simulink model "irp_2018b"  (R2018b)
settings: Solver=VariableStepAuto  StartTime=0.0  StopTime=inf  RelTol=1e-3
libraries: simulink x10, simulink_extras x8
settings Model: Creator=Bartlomiej Mroz  LastModifiedBy=Bartlomiej Mroz

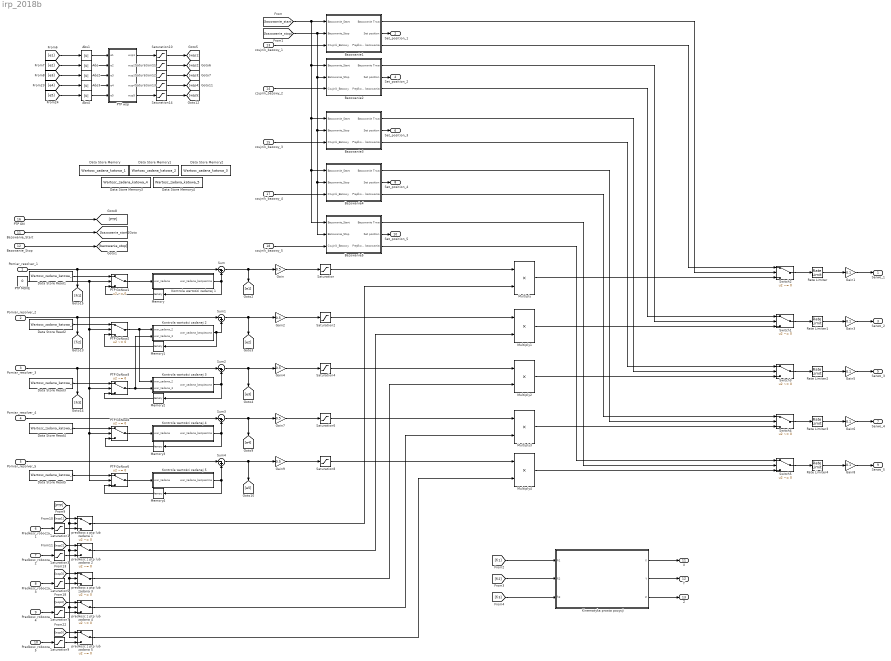
== system irp_2018b ==
  Pomiar_resolver_1 : Inport
  Pomiar_resolver_2 : Inport  Port=2
  Pomiar_resolver_3 : Inport  Port=3
  Pomiar_resolver_4 : Inport  Port=4
  Pomiar_resolver_5 : Inport  Port=5
  Predkosc_robocza_1 : Inport  Port=6
  Predkosc_robocza_2 : Inport  Port=7
  Predkosc_robocza_3 : Inport  Port=8
  Predkosc_robocza_4 : Inport  Port=9
  Predkosc_robocza_5 : Inport  Port=10
  Bazowanie_Start : Inport  Port=11
  Bazowanie_Stop : Inport  Port=12
  czujnik_bazowy_1 : Inport  Port=13
  czujnik_bazowy_2 : Inport  Port=14
  czujnik_bazowy_3 : Inport  Port=15
  PTP ON : Inport  Port=16
  czujnik_bazowy_4 : Inport  Port=17
  czujnik_bazowy_5 : Inport  Port=18
  Abs{,1..4} (5 alike) : Abs
  Bazowanie1 : Subsystem
  Bazowanie2 : Subsystem
  Bazowanie3 : Subsystem
  Bazowanie4 : Subsystem
  Bazowanie5 : Subsystem
  Data Store Memory : DataStoreMemory  DataStoreName=Wartosc_zadana_katowa_1  ReadBeforeWriteMsg=warning  WriteAfterWriteMsg=warning  WriteAfterReadMsg=warning  ShowAdditionalParam=off
  Data Store Memory1 : DataStoreMemory  DataStoreName=Wartosc_zadana_katowa_2  ReadBeforeWriteMsg=warning  WriteAfterWriteMsg=warning  WriteAfterReadMsg=warning  ShowAdditionalParam=off
  Data Store Memory2 : DataStoreMemory  DataStoreName=Wartosc_zadana_katowa_3  ReadBeforeWriteMsg=warning  WriteAfterWriteMsg=warning  WriteAfterReadMsg=warning  ShowAdditionalParam=off
  Data Store Memory3 : DataStoreMemory  DataStoreName=Wartosc_zadana_katowa_4  ReadBeforeWriteMsg=warning  WriteAfterWriteMsg=warning  WriteAfterReadMsg=warning  ShowAdditionalParam=off
  Data Store Memory4 : DataStoreMemory  DataStoreName=Wartosc_zadana_katowa_5  ReadBeforeWriteMsg=warning  WriteAfterWriteMsg=warning  WriteAfterReadMsg=warning  ShowAdditionalParam=off
  Data Store Read1 : DataStoreRead  DataStoreName=Wartosc_zadana_katowa_1
  Data Store Read2 : DataStoreRead  DataStoreName=Wartosc_zadana_katowa_2
  Data Store Read3 : DataStoreRead  DataStoreName=Wartosc_zadana_katowa_3
  Data Store Read4 : DataStoreRead  DataStoreName=Wartosc_zadana_katowa_4
  Data Store Read5 : DataStoreRead  DataStoreName=Wartosc_zadana_katowa_5
  Gain{,2,4,7,9} (5 alike) : Gain  Gain=0.5
  Gain{1,3,5..6,8} (5 alike) : Gain  Gain=0.1
  Kinematyka prosta pozycji : Subsystem
  "Kontrola wartości zadanej 1 " : Subsystem
  Kontrola wartości zadanej 2 : Subsystem
  Kontrola wartości zadanej 3 : Subsystem
  Kontrola wartości zadanej 4 : Subsystem
  Kontrola wartości zadanej 5 : Subsystem
  Memory{,1..4} (5 alike) : Memory
  Multiply{,1..4} (5 alike) : Product
  PTP GoNow{1..5} (5 alike) : Switch  Criteria=u2 ~= 0
  PTP MOVE : Constant  Value=0
  "PTP wsp " : MATLAB Function  TreatAsAtomicUnit=on
  Rate Limiter{,1..4} (5 alike) : RateLimiter  RisingSlewLimit=50  FallingSlewLimit=-50  SampleTimeMode=inherited
  Saturation{,2,4,6,8} (5 alike) : Saturate  UpperLimit=3  LowerLimit=-3
  Saturation{1,3,5,7,9} (5 alike) : Saturate  UpperLimit=1  LowerLimit=0.05
  Saturation{10..14} (5 alike) : Saturate  UpperLimit=1  LowerLimit=0
  Sum{,1..4} (5 alike) : Sum  Inputs=|-+
  Switch{1..5} (5 alike) : Switch  Criteria=u2 ~= 0
  predkosc z ptp lub zadana {1..5} (5 alike) : Switch  Criteria=u2 ~= 0
  Serwo_1 : Outport
  Set_position_1 : Outport  Port=2  VectorParamsAs1DForOutWhenUnconnected=on
  Serwo_2 : Outport  Port=3
  Set_position_2 : Outport  Port=4  VectorParamsAs1DForOutWhenUnconnected=on
  Serwo_3 : Outport  Port=5
  Set_position_3 : Outport  Port=6  VectorParamsAs1DForOutWhenUnconnected=on
  Serwo_4 : Outport  Port=7
  Set_position_4 : Outport  Port=8  VectorParamsAs1DForOutWhenUnconnected=on
  Serwo_5 : Outport  Port=9
  Set_position_5 : Outport  Port=10  VectorParamsAs1DForOutWhenUnconnected=on
  X : Outport  Port=11
  Y : Outport  Port=12
  Z : Outport  Port=13
  wires:
  Pomiar_resolver_1/1 -> Sum/1, [fi1]
  PTP GoNow1/1 -> "Kontrola wartości zadanej 1 "/1(war_zadana)
  "Kontrola wartości zadanej 1 "/1(war_zadana_bezpieczna) -> Sum/2, Memory/1
  Memory/1 -> PTP GoNow1/3
  Data Store Read1/1 -> PTP GoNow1/1
  Sum/1 -> Gain/1, [e1]
  Gain/1 -> Saturation/1
  Rate Limiter/1 -> Gain1/1
  Gain1/1 -> Serwo_1/1
  Saturation/1 -> Multiply/1
  Predkosc_robocza_1/1 -> Saturation1/1
  Bazowanie1/2("Set position ") -> Set_position_1/1
  Multiply/1 -> Switch2/3
  Bazowanie1/1("Bazowanie Trwa ") -> Switch2/2
  Bazowanie1/3(Prędkość bazowania) -> Switch2/1
  Switch2/1 -> Rate Limiter/1
  Bazowanie_Start/1 -> [bazowanie_start]
  Bazowanie_Stop/1 -> [bazowanie_stop]
  [bazowanie_start] -> Bazowanie5/1(Bazowanie_Start), Bazowanie4/1(Bazowanie_Start), Bazowanie3/1(Bazowanie_Start), Bazowanie2/1(Bazowanie_Start), Bazowanie1/1(Bazowanie_Start)
  [bazowanie_stop] -> Bazowanie5/2("Bazowanie_Stop "), Bazowanie4/2("Bazowanie_Stop "), Bazowanie3/2("Bazowanie_Stop "), Bazowanie2/2("Bazowanie_Stop "), Bazowanie1/2("Bazowanie_Stop ")
  czujnik_bazowy_1/1 -> Bazowanie1/3(Czujnik_Bazowy)
  Pomiar_resolver_2/1 -> [fi2], Sum1/1
  czujnik_bazowy_2/1 -> Bazowanie2/3(Czujnik_Bazowy)
  Saturation3/1 -> predkosc z ptp lub zadana 2/3
  Bazowanie2/3(Prędkość bazowania) -> Switch1/1
  Bazowanie2/1("Bazowanie Trwa ") -> Switch1/2
  Predkosc_robocza_2/1 -> Saturation3/1
  Saturation2/1 -> Multiply1/1
  Multiply1/1 -> Switch1/3
  Switch1/1 -> Rate Limiter1/1
  Sum1/1 -> [e2], Gain2/1
  Gain3/1 -> Serwo_2/1
  Kontrola wartości zadanej 2/1(war_zadana_bezpieczna) -> Sum1/2, Memory1/1
  Memory1/1 -> PTP GoNow2/3
  Gain2/1 -> Saturation2/1
  Data Store Read2/1 -> PTP GoNow2/1
  PTP GoNow2/1 -> Kontrola wartości zadanej 3/1(war_zadana_2), Kontrola wartości zadanej 2/1(war_zadana_2)
  Rate Limiter1/1 -> Gain3/1
  Bazowanie2/2("Set position ") -> Set_position_2/1
  Bazowanie3/3(Prędkość bazowania) -> Switch3/1
  Bazowanie3/1("Bazowanie Trwa ") -> Switch3/2
  Saturation4/1 -> Multiply2/1
  Rate Limiter2/1 -> Gain5/1
  PTP GoNow3/1 -> Kontrola wartości zadanej 3/2(war_zadana_3), Kontrola wartości zadanej 2/2(war_zadana_3)
  Multiply2/1 -> Switch3/3
  czujnik_bazowy_3/1 -> Bazowanie3/3(Czujnik_Bazowy)
  Data Store Read3/1 -> PTP GoNow3/1
  Pomiar_resolver_3/1 -> [fi3], Sum2/1
  Predkosc_robocza_3/1 -> Saturation5/1
  Switch3/1 -> Rate Limiter2/1
  Bazowanie3/2("Set position ") -> Set_position_3/1
  Sum2/1 -> Gain4/1, [e3]
  PTP MOVE/1 -> PTP GoNow3/2, PTP GoNow5/2, PTP GoNow4/2, PTP GoNow2/2, PTP GoNow1/2
  Gain5/1 -> Serwo_3/1
  Memory2/1 -> PTP GoNow3/3
  Gain4/1 -> Saturation4/1
  Kontrola wartości zadanej 3/1(war_zadana_bezpieczna) -> Memory2/1, Sum2/2
  predkosc z ptp lub zadana 1/1 -> Multiply/2
  Saturation1/1 -> predkosc z ptp lub zadana 1/3
  PTP ON/1 -> [PTP]
  [PTP] -> predkosc z ptp lub zadana 1/2, predkosc z ptp lub zadana 5/2, predkosc z ptp lub zadana 4/2, predkosc z ptp lub zadana 3/2, predkosc z ptp lub zadana 2/2
  [wsp1] -> predkosc z ptp lub zadana 1/1
  [wsp2] -> predkosc z ptp lub zadana 2/1
  predkosc z ptp lub zadana 2/1 -> Multiply1/2
  [wsp3] -> predkosc z ptp lub zadana 3/1
  Saturation5/1 -> predkosc z ptp lub zadana 3/3
  predkosc z ptp lub zadana 3/1 -> Multiply2/2
  Bazowanie4/2("Set position ") -> Set_position_4/1
  czujnik_bazowy_4/1 -> Bazowanie4/3(Czujnik_Bazowy)
  Bazowanie4/1("Bazowanie Trwa ") -> Switch4/2
  Bazowanie4/3(Prędkość bazowania) -> Switch4/1
  Gain6/1 -> Serwo_4/1
  Rate Limiter3/1 -> Gain6/1
  Switch4/1 -> Rate Limiter3/1
  Multiply3/1 -> Switch4/3
  [e3] -> Abs2/1
  [e2] -> Abs/1
  [e1] -> Abs1/1
  Saturation6/1 -> Multiply3/1
  Gain7/1 -> Saturation6/1
  Sum3/1 -> Gain7/1, [e4]
  Saturation7/1 -> predkosc z ptp lub zadana 4/3
  [wsp4] -> predkosc z ptp lub zadana 4/1
  predkosc z ptp lub zadana 4/1 -> Multiply3/2
  Predkosc_robocza_4/1 -> Saturation7/1
  Pomiar_resolver_4/1 -> Sum3/1
  PTP GoNow4/1 -> Kontrola wartości zadanej 4/1(war_zadana)
  Data Store Read4/1 -> PTP GoNow4/1
  Kontrola wartości zadanej 4/1(war_zadana_bezpieczna) -> Memory3/1, Sum3/2
  Memory3/1 -> PTP GoNow4/3
  czujnik_bazowy_5/1 -> Bazowanie5/3(Czujnik_Bazowy)
  Bazowanie5/2("Set position ") -> Set_position_5/1
  Switch5/1 -> Rate Limiter4/1
  Rate Limiter4/1 -> Gain8/1
  Gain8/1 -> Serwo_5/1
  Bazowanie5/3(Prędkość bazowania) -> Switch5/1
  Bazowanie5/1("Bazowanie Trwa ") -> Switch5/2
  Multiply4/1 -> Switch5/3
  Saturation8/1 -> Multiply4/1
  Gain9/1 -> Saturation8/1
  Sum4/1 -> Gain9/1, [e5]
  predkosc z ptp lub zadana 5/1 -> Multiply4/2
  [wsp5] -> predkosc z ptp lub zadana 5/1
  Saturation9/1 -> predkosc z ptp lub zadana 5/3
  Kontrola wartości zadanej 5/1(war_zadana_bezpieczna) -> Sum4/2, Memory4/1
  PTP GoNow5/1 -> Kontrola wartości zadanej 5/1(war_zadana)
  Memory4/1 -> PTP GoNow5/3
  Pomiar_resolver_5/1 -> Sum4/1
  Predkosc_robocza_5/1 -> Saturation9/1
  Data Store Read5/1 -> PTP GoNow5/1
  Abs4/1 -> "PTP wsp "/5(e5)
  Abs3/1 -> "PTP wsp "/4(e4)
  Abs2/1 -> "PTP wsp "/3(e3)
  Abs/1 -> "PTP wsp "/2(e2)
  Abs1/1 -> "PTP wsp "/1(e1)
  [e4] -> Abs3/1
  [e5] -> Abs4/1
  "PTP wsp "/1(wsp1) -> Saturation10/1
  "PTP wsp "/2(wsp2) -> Saturation11/1
  "PTP wsp "/3(wsp3) -> Saturation12/1
  "PTP wsp "/4(wsp4) -> Saturation13/1
  "PTP wsp "/5(wsp5) -> Saturation14/1
  Saturation10/1 -> [wsp1]
  Saturation11/1 -> [wsp2]
  Saturation12/1 -> [wsp3]
  Saturation13/1 -> [wsp4]
  Saturation14/1 -> [wsp5]
  [fi3] -> Kinematyka prosta pozycji/3("fi3 ")
  [fi2] -> Kinematyka prosta pozycji/2(fi2)
  [fi1] -> Kinematyka prosta pozycji/1(fi1)
  Kinematyka prosta pozycji/1(X) -> X/1
  Kinematyka prosta pozycji/2(Y) -> Y/1
  Kinematyka prosta pozycji/3(Z) -> Z/1

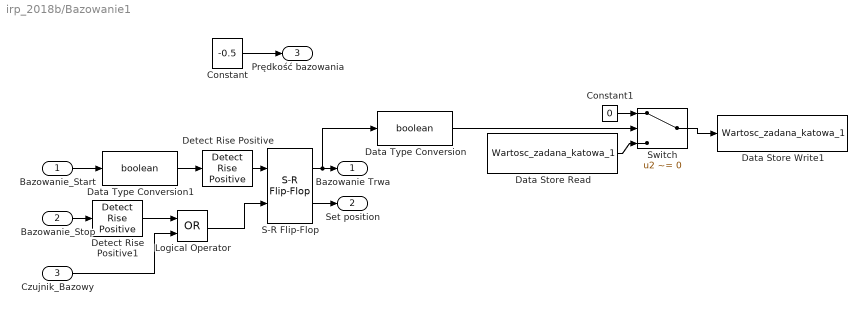
== system irp_2018b/Bazowanie1 ==
  Bazowanie_Start : Inport
  "Bazowanie_Stop " : Inport  Port=2
  Czujnik_Bazowy : Inport  Port=3
  Constant : Constant  Value=-0.5
  Constant1 : Constant  Value=0
  Data Store Read : DataStoreRead  DataStoreName=Wartosc_zadana_katowa_1
  Data Store Write1 : DataStoreWrite  DataStoreName=Wartosc_zadana_katowa_1
  Data Type Conversion : DataTypeConversion  OutDataTypeStr=boolean
  Data Type Conversion1 : DataTypeConversion  OutDataTypeStr=boolean
  Detect Rise Positive : simulink/Logic and Bit Operations/Detect Rise Positive  vinit=0  OutDataTypeStr=boolean
  Detect Rise Positive1 : simulink/Logic and Bit Operations/Detect Rise Positive  vinit=0  OutDataTypeStr=boolean
  Logical Operator : Logic  Operator=OR  AllPortsSameDT=off  OutDataTypeStr=boolean
  S-R Flip-Flop : simulink_extras/Flip Flops/S-R Flip-Flop  initial_condition=0
  Switch : Switch  Criteria=u2 ~= 0
  "Bazowanie Trwa " : Outport
  "Set position " : Outport  Port=2
  Prędkość bazowania : Outport  Port=3
  wires:
  "Bazowanie_Stop "/1 -> Detect Rise Positive1/1
  Czujnik_Bazowy/1 -> Logical Operator/2
  Logical Operator/1 -> S-R Flip-Flop/2
  Bazowanie_Start/1 -> Data Type Conversion1/1
  S-R Flip-Flop/1 -> Data Type Conversion/1, "Bazowanie Trwa "/1
  S-R Flip-Flop/2 -> "Set position "/1
  Constant/1 -> Prędkość bazowania/1
  Switch/1 -> Data Store Write1/1
  Constant1/1 -> Switch/1
  Data Store Read/1 -> Switch/3
  Data Type Conversion/1 -> Switch/2
  Detect Rise Positive1/1 -> Logical Operator/1
  Data Type Conversion1/1 -> Detect Rise Positive/1
  Detect Rise Positive/1 -> S-R Flip-Flop/1

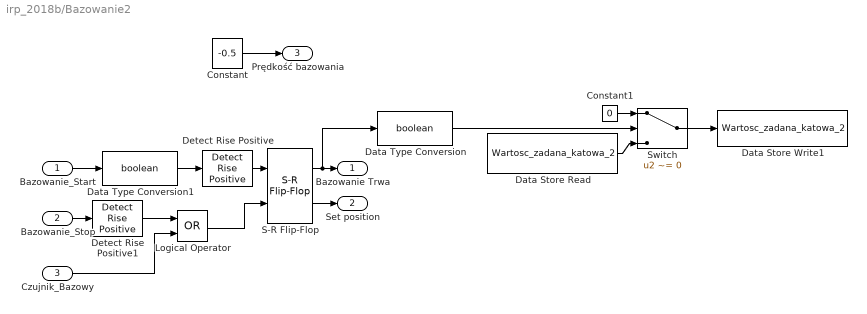
== system irp_2018b/Bazowanie2 ==
  Bazowanie_Start : Inport
  "Bazowanie_Stop " : Inport  Port=2
  Czujnik_Bazowy : Inport  Port=3
  Constant : Constant  Value=-0.5
  Constant1 : Constant  Value=0
  Data Store Read : DataStoreRead  DataStoreName=Wartosc_zadana_katowa_2
  Data Store Write1 : DataStoreWrite  DataStoreName=Wartosc_zadana_katowa_2
  Data Type Conversion : DataTypeConversion  OutDataTypeStr=boolean
  Data Type Conversion1 : DataTypeConversion  OutDataTypeStr=boolean
  Detect Rise Positive : simulink/Logic and Bit Operations/Detect Rise Positive  vinit=0  OutDataTypeStr=boolean
  Detect Rise Positive1 : simulink/Logic and Bit Operations/Detect Rise Positive  vinit=0  OutDataTypeStr=boolean
  Logical Operator : Logic  Operator=OR  AllPortsSameDT=off  OutDataTypeStr=boolean
  S-R Flip-Flop : simulink_extras/Flip Flops/S-R Flip-Flop  initial_condition=0
  Switch : Switch  Criteria=u2 ~= 0
  "Bazowanie Trwa " : Outport
  "Set position " : Outport  Port=2
  Prędkość bazowania : Outport  Port=3
  wires:
  "Bazowanie_Stop "/1 -> Detect Rise Positive1/1
  Czujnik_Bazowy/1 -> Logical Operator/2
  Logical Operator/1 -> S-R Flip-Flop/2
  Bazowanie_Start/1 -> Data Type Conversion1/1
  S-R Flip-Flop/1 -> Data Type Conversion/1, "Bazowanie Trwa "/1
  S-R Flip-Flop/2 -> "Set position "/1
  Constant/1 -> Prędkość bazowania/1
  Switch/1 -> Data Store Write1/1
  Constant1/1 -> Switch/1
  Data Store Read/1 -> Switch/3
  Data Type Conversion/1 -> Switch/2
  Detect Rise Positive1/1 -> Logical Operator/1
  Data Type Conversion1/1 -> Detect Rise Positive/1
  Detect Rise Positive/1 -> S-R Flip-Flop/1

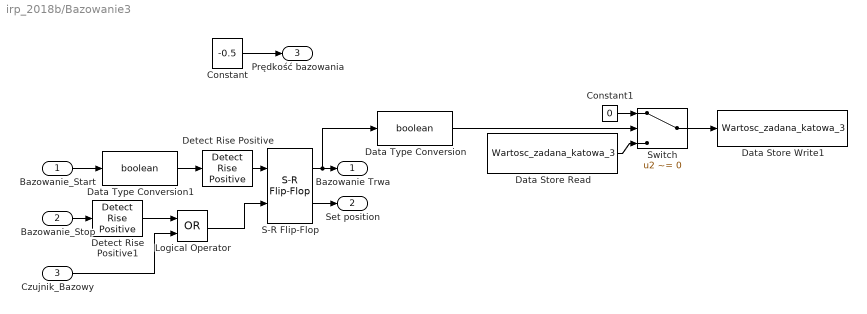
== system irp_2018b/Bazowanie3 ==
  Bazowanie_Start : Inport
  "Bazowanie_Stop " : Inport  Port=2
  Czujnik_Bazowy : Inport  Port=3
  Constant : Constant  Value=-0.5
  Constant1 : Constant  Value=0
  Data Store Read : DataStoreRead  DataStoreName=Wartosc_zadana_katowa_3
  Data Store Write1 : DataStoreWrite  DataStoreName=Wartosc_zadana_katowa_3
  Data Type Conversion : DataTypeConversion  OutDataTypeStr=boolean
  Data Type Conversion1 : DataTypeConversion  OutDataTypeStr=boolean
  Detect Rise Positive : simulink/Logic and Bit Operations/Detect Rise Positive  vinit=0  OutDataTypeStr=boolean
  Detect Rise Positive1 : simulink/Logic and Bit Operations/Detect Rise Positive  vinit=0  OutDataTypeStr=boolean
  Logical Operator : Logic  Operator=OR  AllPortsSameDT=off  OutDataTypeStr=boolean
  S-R Flip-Flop : simulink_extras/Flip Flops/S-R Flip-Flop  initial_condition=0
  Switch : Switch  Criteria=u2 ~= 0
  "Bazowanie Trwa " : Outport
  "Set position " : Outport  Port=2
  Prędkość bazowania : Outport  Port=3
  wires:
  "Bazowanie_Stop "/1 -> Detect Rise Positive1/1
  Czujnik_Bazowy/1 -> Logical Operator/2
  Logical Operator/1 -> S-R Flip-Flop/2
  Bazowanie_Start/1 -> Data Type Conversion1/1
  S-R Flip-Flop/1 -> Data Type Conversion/1, "Bazowanie Trwa "/1
  S-R Flip-Flop/2 -> "Set position "/1
  Constant/1 -> Prędkość bazowania/1
  Switch/1 -> Data Store Write1/1
  Constant1/1 -> Switch/1
  Data Store Read/1 -> Switch/3
  Data Type Conversion/1 -> Switch/2
  Detect Rise Positive1/1 -> Logical Operator/1
  Data Type Conversion1/1 -> Detect Rise Positive/1
  Detect Rise Positive/1 -> S-R Flip-Flop/1

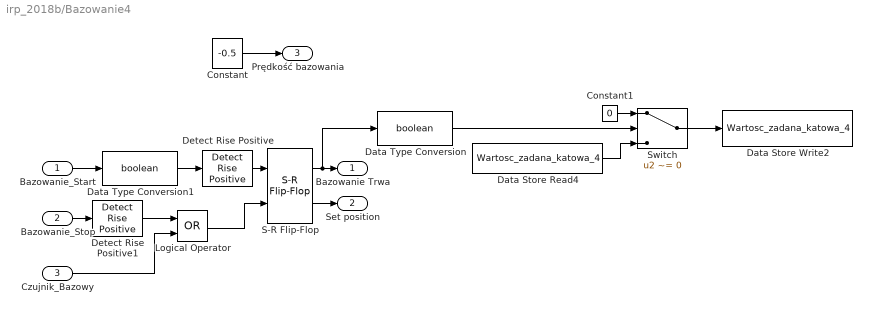
== system irp_2018b/Bazowanie4 ==
  Bazowanie_Start : Inport
  "Bazowanie_Stop " : Inport  Port=2
  Czujnik_Bazowy : Inport  Port=3
  Constant : Constant  Value=-0.5
  Constant1 : Constant  Value=0
  Data Store Read4 : DataStoreRead  DataStoreName=Wartosc_zadana_katowa_4
  Data Store Write2 : DataStoreWrite  DataStoreName=Wartosc_zadana_katowa_4
  Data Type Conversion : DataTypeConversion  OutDataTypeStr=boolean
  Data Type Conversion1 : DataTypeConversion  OutDataTypeStr=boolean
  Detect Rise Positive : simulink/Logic and Bit Operations/Detect Rise Positive  vinit=0  OutDataTypeStr=boolean
  Detect Rise Positive1 : simulink/Logic and Bit Operations/Detect Rise Positive  vinit=0  OutDataTypeStr=boolean
  Logical Operator : Logic  Operator=OR  AllPortsSameDT=off  OutDataTypeStr=boolean
  S-R Flip-Flop : simulink_extras/Flip Flops/S-R Flip-Flop  initial_condition=0
  Switch : Switch  Criteria=u2 ~= 0
  "Bazowanie Trwa " : Outport
  "Set position " : Outport  Port=2
  Prędkość bazowania : Outport  Port=3
  wires:
  Detect Rise Positive/1 -> S-R Flip-Flop/1
  Data Type Conversion1/1 -> Detect Rise Positive/1
  Detect Rise Positive1/1 -> Logical Operator/1
  Data Type Conversion/1 -> Switch/2
  Data Store Read4/1 -> Switch/3
  Constant1/1 -> Switch/1
  Switch/1 -> Data Store Write2/1
  Constant/1 -> Prędkość bazowania/1
  S-R Flip-Flop/2 -> "Set position "/1
  S-R Flip-Flop/1 -> "Bazowanie Trwa "/1, Data Type Conversion/1
  Bazowanie_Start/1 -> Data Type Conversion1/1
  Logical Operator/1 -> S-R Flip-Flop/2
  Czujnik_Bazowy/1 -> Logical Operator/2
  "Bazowanie_Stop "/1 -> Detect Rise Positive1/1

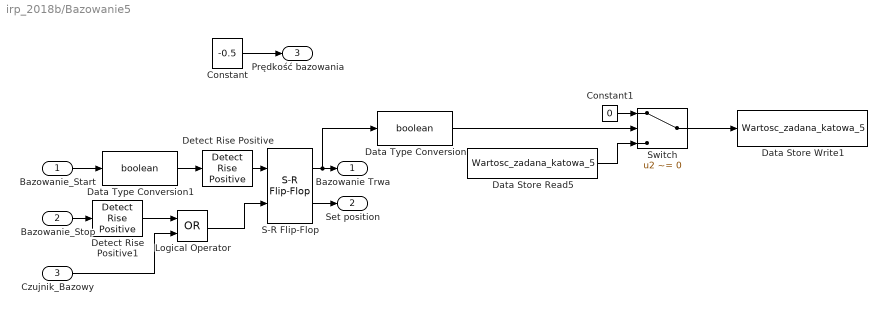
== system irp_2018b/Bazowanie5 ==
  Bazowanie_Start : Inport
  "Bazowanie_Stop " : Inport  Port=2
  Czujnik_Bazowy : Inport  Port=3
  Constant : Constant  Value=-0.5
  Constant1 : Constant  Value=0
  Data Store Read5 : DataStoreRead  DataStoreName=Wartosc_zadana_katowa_5
  Data Store Write1 : DataStoreWrite  DataStoreName=Wartosc_zadana_katowa_5
  Data Type Conversion : DataTypeConversion  OutDataTypeStr=boolean
  Data Type Conversion1 : DataTypeConversion  OutDataTypeStr=boolean
  Detect Rise Positive : simulink/Logic and Bit Operations/Detect Rise Positive  vinit=0  OutDataTypeStr=boolean
  Detect Rise Positive1 : simulink/Logic and Bit Operations/Detect Rise Positive  vinit=0  OutDataTypeStr=boolean
  Logical Operator : Logic  Operator=OR  AllPortsSameDT=off  OutDataTypeStr=boolean
  S-R Flip-Flop : simulink_extras/Flip Flops/S-R Flip-Flop  initial_condition=0
  Switch : Switch  Criteria=u2 ~= 0
  "Bazowanie Trwa " : Outport
  "Set position " : Outport  Port=2
  Prędkość bazowania : Outport  Port=3
  wires:
  "Bazowanie_Stop "/1 -> Detect Rise Positive1/1
  Czujnik_Bazowy/1 -> Logical Operator/2
  Logical Operator/1 -> S-R Flip-Flop/2
  Bazowanie_Start/1 -> Data Type Conversion1/1
  S-R Flip-Flop/1 -> Data Type Conversion/1, "Bazowanie Trwa "/1
  S-R Flip-Flop/2 -> "Set position "/1
  Constant/1 -> Prędkość bazowania/1
  Switch/1 -> Data Store Write1/1
  Constant1/1 -> Switch/1
  Data Store Read5/1 -> Switch/3
  Data Type Conversion/1 -> Switch/2
  Detect Rise Positive1/1 -> Logical Operator/1
  Data Type Conversion1/1 -> Detect Rise Positive/1
  Detect Rise Positive/1 -> S-R Flip-Flop/1

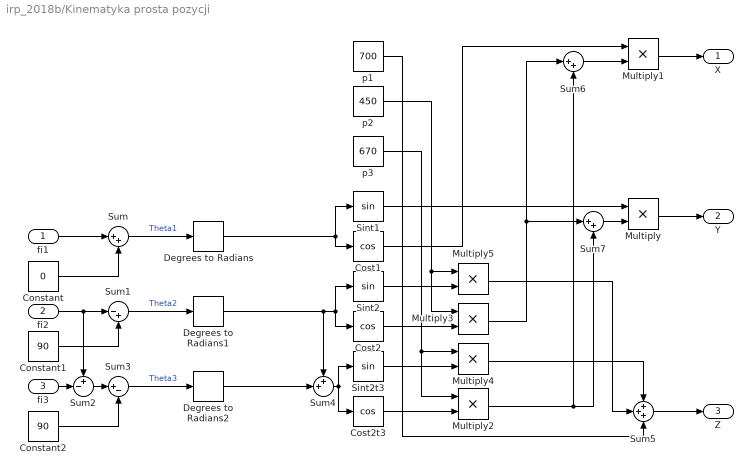
== system irp_2018b/Kinematyka prosta pozycji ==
  fi1 : Inport
  fi2 : Inport  Port=2
  "fi3 " : Inport  Port=3
  Constant : Constant  Value=0
  Constant1 : Constant  Value=90
  Constant2 : Constant  Value=90
  Cost1 : Trigonometry  Operator=cos
  Cost2 : Trigonometry  Operator=cos
  Cost2t3 : Trigonometry  Operator=cos
  Degrees to Radians : simulink_extras/Transformations/Degrees to Radians
  Degrees to Radians1 : simulink_extras/Transformations/Degrees to Radians
  Degrees to Radians2 : simulink_extras/Transformations/Degrees to Radians
  Multiply{,1..5} (6 alike) : Product
  Sint1 : Trigonometry
  Sint2 : Trigonometry
  Sint2t3 : Trigonometry
  Sum : Sum  Inputs=|++
  Sum1 : Sum  Inputs=|-+
  Sum2 : Sum  Inputs=+-|
  Sum3 : Sum  Inputs=|+-
  Sum4 : Sum  Inputs=++|
  Sum5 : Sum  Inputs=+++
  Sum6 : Sum  Inputs=|++
  Sum7 : Sum  Inputs=|++
  p1 : Constant  Value=700
  p2 : Constant  Value=450
  p3 : Constant  Value=670
  X : Outport
  Y : Outport  Port=2
  Z : Outport  Port=3
  wires:
  fi1/1 -> Sum/1
  Constant/1 -> Sum/2
  Sum/1 -> Degrees to Radians/1  "Theta1"
  fi2/1 -> Sum2/1, Sum1/1
  Constant1/1 -> Sum1/2
  Sum1/1 -> Degrees to Radians1/1  "Theta2"
  "fi3 "/1 -> Sum2/2
  Sum2/1 -> Sum3/1
  Sum3/1 -> Degrees to Radians2/1  "Theta3"
  Constant2/1 -> Sum3/2
  Sum4/1 -> Cost2t3/1, Sint2t3/1
  Degrees to Radians1/1 -> Cost2/1, Sint2/1, Sum4/1
  Degrees to Radians2/1 -> Sum4/2
  Degrees to Radians/1 -> Cost1/1, Sint1/1
  Sum5/1 -> Z/1
  Multiply/1 -> Y/1
  Multiply1/1 -> X/1
  Cost1/1 -> Multiply1/1
  Sum6/1 -> Multiply1/2
  Cost2t3/1 -> Multiply2/2
  Cost2/1 -> Multiply3/2
  p3/1 -> Multiply4/1, Multiply2/1
  p2/1 -> Multiply5/1, Multiply3/1
  Multiply3/1 -> Sum7/1, Sum6/1
  Multiply2/1 -> Sum7/2, Sum6/2
  Sum7/1 -> Multiply/2
  Sint1/1 -> Multiply/1
  Sint2t3/1 -> Multiply4/2
  Multiply4/1 -> Sum5/1
  Sint2/1 -> Multiply5/2
  Multiply5/1 -> Sum5/2
  p1/1 -> Sum5/3

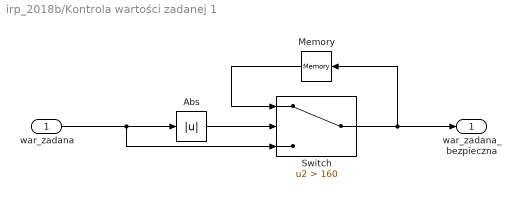
== system irp_2018b/Kontrola wartości zadanej 1  ==
  war_zadana : Inport
  Abs : Abs
  Memory : Memory
  Switch : Switch  Criteria=u2 > Threshold  Threshold=160
  war_zadana_bezpieczna : Outport
  wires:
  war_zadana/1 -> Switch/3, Abs/1
  Abs/1 -> Switch/2
  Switch/1 -> Memory/1, war_zadana_bezpieczna/1
  Memory/1 -> Switch/1

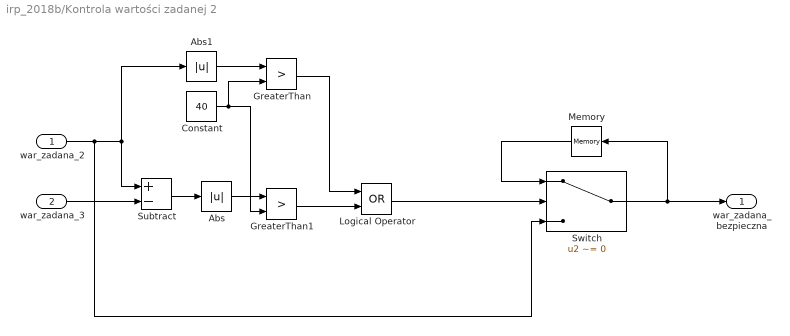
== system irp_2018b/Kontrola wartości zadanej 2 ==
  war_zadana_2 : Inport
  war_zadana_3 : Inport  Port=2
  Abs : Abs
  Abs1 : Abs
  Constant : Constant  Value=40
  GreaterThan : RelationalOperator  Operator=>  OutDataTypeStr=boolean  RndMeth=Simplest
  GreaterThan1 : RelationalOperator  Operator=>  OutDataTypeStr=boolean  RndMeth=Simplest
  Logical Operator : Logic  Operator=OR  AllPortsSameDT=off  OutDataTypeStr=boolean
  Memory : Memory
  Subtract : Sum  Inputs=+-
  Switch : Switch  Criteria=u2 ~= 0  Threshold=40
  war_zadana_bezpieczna : Outport
  wires:
  Switch/1 -> Memory/1, war_zadana_bezpieczna/1
  Memory/1 -> Switch/1
  war_zadana_2/1 -> Abs1/1, Subtract/1, Switch/3
  war_zadana_3/1 -> Subtract/2
  Subtract/1 -> Abs/1
  Abs1/1 -> GreaterThan/1
  Constant/1 -> GreaterThan1/2, GreaterThan/2
  Abs/1 -> GreaterThan1/1
  GreaterThan/1 -> Logical Operator/1
  GreaterThan1/1 -> Logical Operator/2
  Logical Operator/1 -> Switch/2

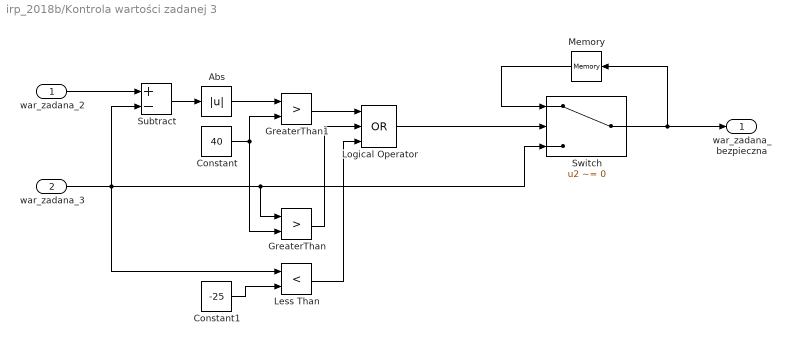
== system irp_2018b/Kontrola wartości zadanej 3 ==
  war_zadana_2 : Inport
  war_zadana_3 : Inport  Port=2
  Abs : Abs
  Constant : Constant  Value=40
  Constant1 : Constant  Value=-25
  GreaterThan : RelationalOperator  Operator=>  OutDataTypeStr=boolean  RndMeth=Simplest
  GreaterThan1 : RelationalOperator  Operator=>  OutDataTypeStr=boolean  RndMeth=Simplest
  Less Than : RelationalOperator  Operator=<  OutDataTypeStr=boolean  RndMeth=Simplest
  Logical Operator : Logic  Operator=OR  Inputs=3  AllPortsSameDT=off  OutDataTypeStr=boolean
  Memory : Memory
  Subtract : Sum  Inputs=+-
  Switch : Switch  Criteria=u2 ~= 0  Threshold=40
  war_zadana_bezpieczna : Outport
  wires:
  Switch/1 -> Memory/1, war_zadana_bezpieczna/1
  Memory/1 -> Switch/1
  war_zadana_2/1 -> Subtract/1
  war_zadana_3/1 -> Less Than/1, Subtract/2, GreaterThan/1, Switch/3
  Subtract/1 -> Abs/1
  Constant/1 -> GreaterThan/2, GreaterThan1/2
  Abs/1 -> GreaterThan1/1
  Logical Operator/1 -> Switch/2
  Constant1/1 -> Less Than/2
  GreaterThan1/1 -> Logical Operator/1
  GreaterThan/1 -> Logical Operator/2
  Less Than/1 -> Logical Operator/3

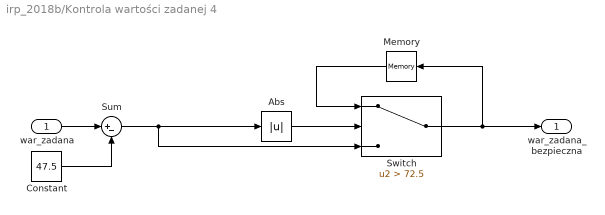
== system irp_2018b/Kontrola wartości zadanej 4 ==
  war_zadana : Inport
  Abs : Abs
  Constant : Constant  Value=47.5
  Memory : Memory
  Sum : Sum  Inputs=|+-
  Switch : Switch  Criteria=u2 > Threshold  Threshold=72.5
  war_zadana_bezpieczna : Outport
  wires:
  Memory/1 -> Switch/1
  Switch/1 -> war_zadana_bezpieczna/1, Memory/1
  Abs/1 -> Switch/2
  Constant/1 -> Sum/2
  Sum/1 -> Switch/3, Abs/1
  war_zadana/1 -> Sum/1

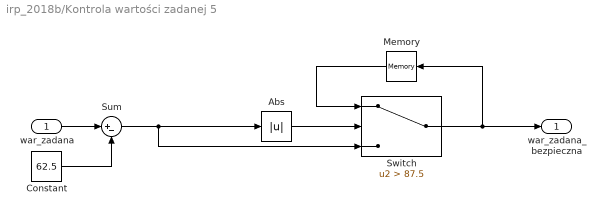
== system irp_2018b/Kontrola wartości zadanej 5 ==
  war_zadana : Inport
  Abs : Abs
  Constant : Constant  Value=62.5
  Memory : Memory
  Sum : Sum  Inputs=|+-
  Switch : Switch  Criteria=u2 > Threshold  Threshold=87.5
  war_zadana_bezpieczna : Outport
  wires:
  war_zadana/1 -> Sum/1
  Sum/1 -> Abs/1, Switch/3
  Constant/1 -> Sum/2
  Abs/1 -> Switch/2
  Switch/1 -> Memory/1, war_zadana_bezpieczna/1
  Memory/1 -> Switch/1

== matlab function irp_2018b/PTP wsp  ==
  data: e1 input; wsp1 output; e2 input; wsp2 output; e3 input; wsp3 output; e4 input; e5 input; wsp4 output; wsp5 output
function [wsp1,wsp2,wsp3,wsp4,wsp5] = fcn(e1,e2,e3,e4,e5)
denum = max(e1,e2,e3);
if ~denum
    denum = 0.01;
end
wsp1 = e1/denum;
wsp2 = e2/denum;
wsp3 = e3/denum;
wsp4 = e4/denum;
wsp5 = e5/denum;
